simulink model "sampleModel1750"  (R2023a)
settings: Solver=VariableStepAuto  StartTime=0.0  StopTime=10.0  RelTol=1e-3
libraries: hdlsllib x5
settings Model: Creator=user1  LastModifiedBy=user1

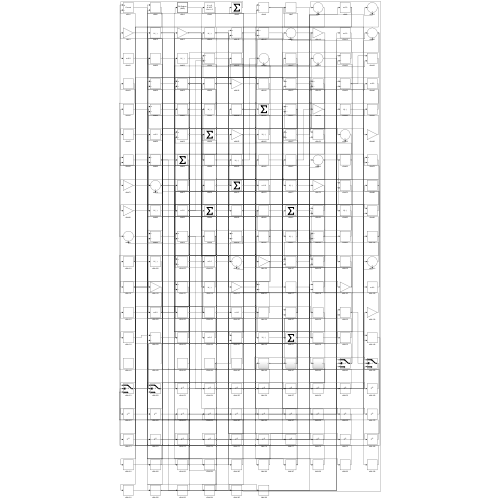
[thumbnail: Simulink's stored preview of the top-level diagram]
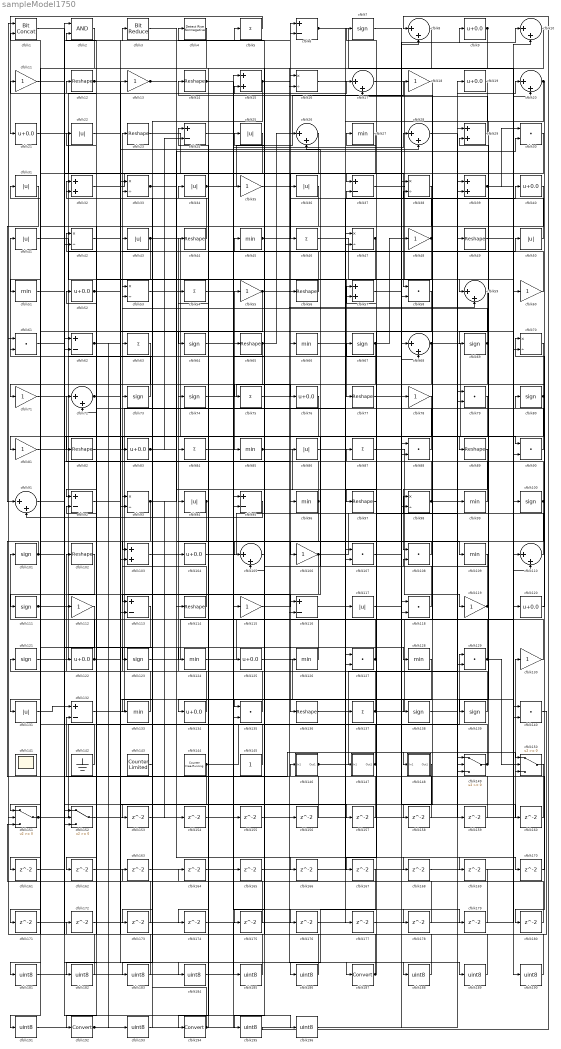
== system sampleModel1750 ==
  cfblk1 : hdlsllib/Logic and Bit Operations/Bit Concat  numInputs=2
  cfblk{8,10,17,20,26,28,59,68,72,91,105,110} (12 alike) : Sum  Inputs=|++
  cfblk{7,64,67,69,73..74,80,100..101,111,121,123,138..139} (14 alike) : Signum
  cfblk{12,14,23,44,49,56,65,77,82,89,97,102,114,136} (14 alike) : Reshape
  cfblk{15,29,32,39,57,103} (6 alike) : Sum
  cfblk{9,19,21,40,52,76,83,104,120,122,125,134} (12 alike) : Bias  Bias=0.0  SaturateOnIntegerOverflow=off
  cfblk{11,13,18,35,48,55,60,71,78,81,106,112,115,119,130} (15 alike) : Gain
  cfblk{30,58,61,79,88,90,107..108,118,127,129,135,140} (13 alike) : DotProduct  OutDataTypeStr=Inherit: Inherit via internal rule
  cfblk{27,45,51,66,85,96,99,109,124,126,128,133} (12 alike) : MinMax
  cfblk{6,24,37,62,92,95,113,116,132} (9 alike) : Sum  Inputs=+-
  cfblk{22,25,31,34,36,41,43,50,86,94,117,131} (12 alike) : Abs  SaturateOnIntegerOverflow=off
  cfblk{5,46,54,63,75,84,87,137} (8 alike) : Sum  Inputs=+
  cfblk141 : Scope
      settings: Floating=on
  cfblk142 : Ground
  cfblk143 : hdlsllib/Sources/Counter Limited  uplimit=7  tsamp=-1
  cfblk144 : hdlsllib/Sources/Counter Free-Running  NumBits=16  tsamp=-1
  cfblk145 : Constant  SampleTime=-1
  cfblk146 : Subsystem
      settings: LibrarySourceBlock=|
      | hdlsllib/Ports &
      | Subsystems/Subsystem
  cfblk147 : Subsystem
      settings: LibrarySourceBlock=|
      | hdlsllib/Ports &
      | Subsystems/Subsystem
  cfblk148 : Subsystem
      settings: LibrarySourceBlock=|
      | hdlsllib/Ports &
      | Subsystems/Subsystem
  cfblk{149..152} (4 alike) : Switch  SaturateOnIntegerOverflow=off  InputSameDT=off
  cfblk{153..180} (28 alike) : Delay  SampleTime=1
  cfblk{16,33,38,42,47,53,70,93,98} (9 alike) : Product  Inputs=*/  RndMeth=Zero  SaturateOnIntegerOverflow=on
  cfblk{181..186,188..191,193,195..196} (13 alike) : DataTypeConversion  OutDataTypeStr=uint8  SaturateOnIntegerOverflow=off  RndMeth=Floor
  cfblk187 : DataTypeConversion  SaturateOnIntegerOverflow=off  RndMeth=Floor
  cfblk192 : DataTypeConversion  SaturateOnIntegerOverflow=off  RndMeth=Floor
  cfblk194 : DataTypeConversion  SaturateOnIntegerOverflow=off  RndMeth=Floor
  cfblk2 : Logic  AllPortsSameDT=off  OutDataTypeStr=boolean
  cfblk3 : hdlsllib/Logic and Bit Operations/Bit Reduce  mode=AND
  cfblk4 : hdlsllib/Logic and Bit Operations/Detect Rise Nonnegative  vinit=0  OutDataTypeStr=boolean
  wires:
  cfblk122/1 -> cfblk101/1, cfblk124/1, cfblk126/1
  cfblk111/1 -> cfblk136/1, cfblk3/1, cfblk86/1
  cfblk129/1 -> cfblk14/1, cfblk150/2
  cfblk115/1 -> cfblk6/1
  cfblk88/1 -> cfblk23/1
  cfblk96/1 -> cfblk53/1, cfblk113/2
  cfblk81/1 -> cfblk50/1
  cfblk17/1 -> cfblk59/1
  cfblk67/1 -> cfblk48/1, cfblk153/1
  cfblk150/1 -> cfblk146/1(In1)
  cfblk131/1 -> cfblk132/1
  cfblk100/1 -> cfblk70/1, cfblk72/1, cfblk173/1
  cfblk87/1 -> cfblk119/1
  cfblk43/1 -> cfblk89/1, cfblk93/2
  cfblk144/1 -> cfblk129/1, cfblk152/2
  cfblk114/1 -> cfblk73/1
  cfblk39/1 -> cfblk60/1, cfblk30/1
  cfblk113/1 -> cfblk121/1
  cfblk84/1 -> cfblk55/1
  cfblk101/1 -> cfblk148/1(In1), cfblk196/1
  cfblk119/1 -> cfblk96/1, cfblk26/2
  cfblk139/1 -> cfblk44/1
  cfblk136/1 -> cfblk78/1
  cfblk20/1 -> cfblk139/1, cfblk180/1
  cfblk137/1 -> cfblk29/1, cfblk122/1
  cfblk14/1 -> cfblk115/1, cfblk178/1
  cfblk121/1 -> cfblk17/1
  cfblk145/1 -> cfblk52/1
  cfblk73/1 -> cfblk41/1
  cfblk118/1 -> cfblk4/1
  cfblk5/1 -> cfblk21/1
  cfblk89/1 -> cfblk108/1
  cfblk127/1 -> cfblk34/1, cfblk7/1
  cfblk125/1 -> cfblk138/1
  cfblk47/1 -> cfblk77/1, cfblk72/2
  cfblk135/1 -> cfblk94/1
  cfblk50/1 -> cfblk16/1
  cfblk94/1 -> cfblk111/1, cfblk133/1
  cfblk44/1 -> cfblk32/1
  cfblk16/1 -> cfblk88/2
  cfblk31/1 -> cfblk91/1
  cfblk142/1 -> cfblk31/1
  cfblk69/1 -> cfblk97/1, cfblk53/2
  cfblk143/1 -> cfblk43/1
  cfblk62/1 -> cfblk82/1, cfblk6/2, cfblk193/1
  cfblk65/1 -> cfblk26/1, cfblk174/1
  cfblk60/1 -> cfblk45/1
  cfblk34/1 -> cfblk18/1, cfblk28/1
  cfblk56/1 -> cfblk24/1
  cfblk107/1 -> cfblk10/1
  cfblk109/1 -> cfblk108/2
  cfblk132/1 -> cfblk47/1
  cfblk36/1 -> cfblk92/1
  cfblk124/1 -> cfblk100/1
  cfblk82/1 -> cfblk56/1
  cfblk128/1 -> cfblk134/1
  cfblk10/1 -> cfblk16/2
  cfblk30/1 -> cfblk64/1
  cfblk147/1(Out1) -> cfblk74/1, cfblk54/1
  cfblk21/1 -> cfblk58/1
  cfblk99/1 -> cfblk22/1
  cfblk27/1 -> cfblk135/1
  cfblk54/1 -> cfblk35/1
  cfblk23/1 -> cfblk46/1
  cfblk8/1 -> cfblk194/1
  cfblk80/1 -> cfblk95/2, cfblk71/1
  cfblk68/1 -> cfblk120/1, cfblk105/2
  cfblk134/1 -> cfblk93/1
  cfblk130/1 -> cfblk42/1
  cfblk3/1 -> cfblk114/1
  cfblk106/1 -> cfblk19/1, cfblk113/1
  cfblk25/1 -> cfblk51/1
  cfblk126/1 -> cfblk65/1
  cfblk133/1 -> cfblk102/1
  cfblk38/1 -> cfblk127/2
  cfblk110/1 -> cfblk67/1
  cfblk52/1 -> cfblk12/1, cfblk28/2
  cfblk104/1 -> cfblk98/1
  cfblk92/1 -> cfblk15/2
  cfblk74/1 -> cfblk76/1
  cfblk9/1 -> cfblk75/1, cfblk62/2
  cfblk63/1 -> cfblk192/1
  cfblk146/1(Out1) -> cfblk39/1, cfblk170/1
  cfblk79/1 -> cfblk131/1
  cfblk152/1 -> cfblk130/1
  cfblk32/1 -> cfblk36/1
  cfblk86/1 -> cfblk117/1
  cfblk77/1 -> cfblk9/1
  cfblk85/1 -> cfblk147/1(In1), cfblk5/1
  cfblk138/1 -> cfblk20/1
  cfblk33/1 -> cfblk106/1, cfblk98/2, cfblk109/1
  cfblk78/1 -> cfblk116/1
  cfblk83/1 -> cfblk105/1, cfblk24/2, cfblk66/1
  cfblk151/1 -> cfblk118/2, cfblk39/2
  cfblk51/1 -> cfblk90/1
  cfblk11/1 -> cfblk37/1
  cfblk59/1 -> cfblk69/1
  cfblk98/1 -> cfblk79/2, cfblk27/1
  cfblk117/1 -> cfblk150/1
  cfblk112/1 -> cfblk151/1
  cfblk123/1 -> cfblk68/2
  cfblk57/1 -> cfblk38/1
  cfblk41/1 -> cfblk85/1
  cfblk97/1 -> cfblk57/1
  cfblk108/1 -> cfblk103/1
  cfblk116/1 -> cfblk40/1
  cfblk13/1 -> cfblk104/1, cfblk57/2
  cfblk55/1 -> cfblk81/1, cfblk188/1
  cfblk93/1 -> cfblk30/2, cfblk152/3, cfblk154/1
  cfblk53/1 -> cfblk116/2
  cfblk90/1 -> cfblk11/1
  cfblk48/1 -> cfblk38/2, cfblk182/1, cfblk183/1
  cfblk120/1 -> cfblk80/1
  cfblk46/1 -> cfblk149/1
  cfblk72/1 -> cfblk135/2, cfblk140/2
  cfblk45/1 -> cfblk168/1, cfblk169/1
  cfblk6/1 -> cfblk137/1, cfblk140/1
  cfblk61/1 -> cfblk187/1
  cfblk35/1 -> cfblk59/2
  cfblk91/1 -> cfblk128/1
  cfblk76/1 -> cfblk103/2
  cfblk26/1 -> cfblk83/1
  cfblk12/1 -> cfblk70/2, cfblk189/1
  cfblk19/1 -> cfblk107/2
  cfblk42/1 -> cfblk13/1
  cfblk37/1 -> cfblk110/2
  cfblk149/1 -> cfblk112/1, cfblk29/2
  cfblk29/1 -> cfblk17/2
  cfblk95/1 -> cfblk91/2
  cfblk15/1 -> cfblk123/1, cfblk179/1
  cfblk71/1 -> cfblk58/2
  cfblk153/1 -> cfblk110/1
  cfblk154/1 -> cfblk20/2
  cfblk64/1 -> cfblk155/1
  cfblk155/1 -> cfblk118/1
  cfblk75/1 -> cfblk156/1
  cfblk156/1 -> cfblk132/2
  cfblk22/1 -> cfblk157/1
  cfblk157/1 -> cfblk107/1
  cfblk18/1 -> cfblk158/1
  cfblk158/1 -> cfblk37/2
  cfblk28/1 -> cfblk159/1
  cfblk159/1 -> cfblk127/1
  cfblk7/1 -> cfblk160/1
  cfblk160/1 -> cfblk92/2
  cfblk40/1 -> cfblk161/1
  cfblk161/1 -> cfblk42/2
  cfblk148/1(Out1) -> cfblk162/1
  cfblk162/1 -> cfblk95/1
  cfblk163/1 -> cfblk15/1
  cfblk164/1 -> cfblk47/2
  cfblk165/1 -> cfblk90/2
  cfblk103/1 -> cfblk166/1
  cfblk166/1 -> cfblk79/1
  cfblk58/1 -> cfblk167/1
  cfblk168/1 -> cfblk149/2
  cfblk169/1 -> cfblk151/3
  cfblk170/1 -> cfblk150/3
  cfblk102/1 -> cfblk171/1
  cfblk171/1 -> cfblk88/1
  cfblk140/1 -> cfblk172/1
  cfblk172/1 -> cfblk68/1
  cfblk173/1 -> cfblk152/1
  cfblk105/1 -> cfblk175/1
  cfblk175/1 -> cfblk62/1
  cfblk24/1 -> cfblk176/1
  cfblk176/1 -> cfblk10/2
  cfblk66/1 -> cfblk177/1
  cfblk177/1 -> cfblk149/3
  cfblk178/1 -> cfblk32/2
  cfblk179/1 -> cfblk33/2
  cfblk180/1 -> cfblk151/2
  cfblk2/1 -> cfblk181/1
  cfblk181/1 -> cfblk125/1
  cfblk182/1 -> cfblk2/1
  cfblk183/1 -> cfblk2/2
  cfblk1/1 -> cfblk184/1
  cfblk184/1 -> cfblk84/1
  cfblk174/1 -> cfblk185/1
  cfblk185/1 -> cfblk1/1
  cfblk167/1 -> cfblk186/1
  cfblk186/1 -> cfblk1/2
  cfblk187/1 -> cfblk87/1, cfblk33/1
  cfblk188/1 -> cfblk61/1
  cfblk189/1 -> cfblk61/2
  cfblk49/1 -> cfblk190/1
  cfblk190/1 -> cfblk25/1
  cfblk4/1 -> cfblk191/1
  cfblk191/1 -> cfblk49/1
  cfblk192/1 -> cfblk129/2, cfblk99/1
  cfblk193/1 -> cfblk63/1
  cfblk194/1 -> cfblk165/1, cfblk164/1, cfblk163/1
  cfblk70/1 -> cfblk195/1
  cfblk195/1 -> cfblk8/1
  cfblk196/1 -> cfblk8/2

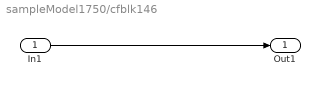
== system sampleModel1750/cfblk146 ==
  In1 : Inport
  Out1 : Outport
  wires:
  In1/1 -> Out1/1

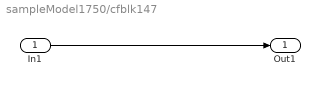
== system sampleModel1750/cfblk147 ==
  In1 : Inport
  Out1 : Outport
  wires:
  In1/1 -> Out1/1

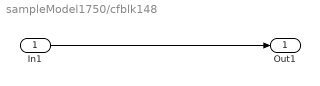
== system sampleModel1750/cfblk148 ==
  In1 : Inport
  Out1 : Outport
  wires:
  In1/1 -> Out1/1
